simulink model "Autopilot_q_full_5may_new1"  (R2020a)
settings: Solver=ode4  StartTime=0.0  StopTime=300  FixedStep=0.01  RelTol=1e-3
undefined symbols (not defined in the file or in its folder): Aero_cofficients, Atmosphere_pert, Atmospheric_model, Counter_sensor_model, Earth, error_global, flags_global, Guidance_Flags_global, INT_global, param_guidance, Payload_data, Plane_state_mode_finish_catcher_ftr_mode, Plane_state_mode_finish_catcher_fw_mode, Plane_state_mode_finish_catcher_q_mode, Plane_state_mode_finish_catcher_rtr_mode, Plane_state_store, propulsion_model, propulsion_model_int, Structural_data, Thrust_data_store, time_global, WGS84, Wind_data, Wind_model_int, Wind_pert_factor
libraries: simulink x33, aerolibactuator x15, cstblocks x3, aerolibatmos2 x2, aerolibfltsims x1, aerolibtransform2 x1, shared6dof x1
(part 2 of 10)

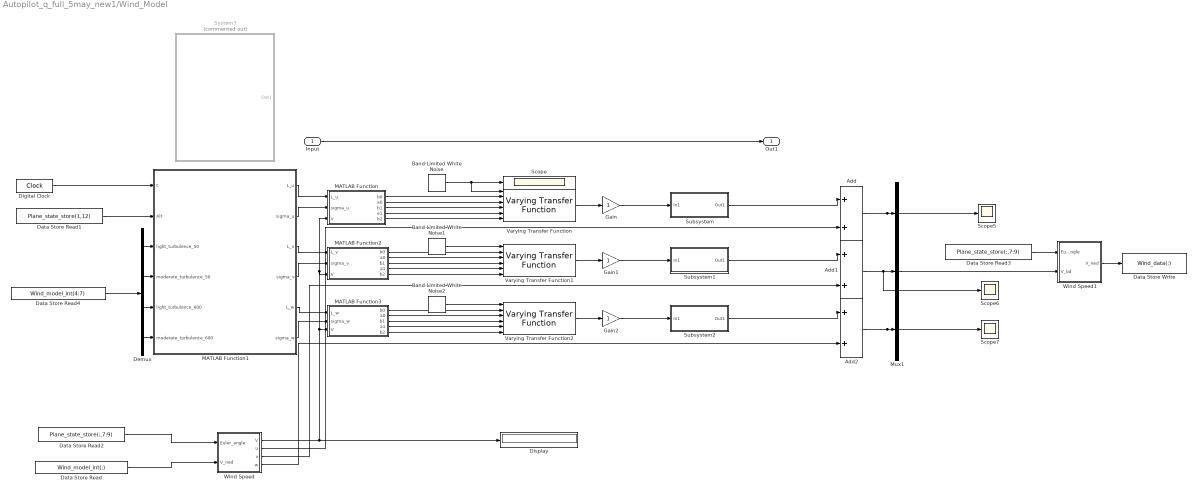
== system Autopilot_q_full_5may_new1/Wind_Model ==
  Input : Inport
  Add : Sum
  Add1 : Sum
  Add2 : Sum
  Band-Limited White Noise : simulink/Sources/Band-Limited White Noise  Cov=[0.001]  Ts=0.01  seed=[23341]
  Band-Limited White Noise1 : simulink/Sources/Band-Limited White Noise  Cov=[0.001]  Ts=0.01  seed=[23341]
  Band-Limited White Noise2 : simulink/Sources/Band-Limited White Noise  Cov=[0.001]  Ts=0.01  seed=[23341]
  Data Store Read : DataStoreRead  DataStoreName=Wind_model_int  SampleTime=0.01  DataStoreElements=Wind_model_int(:)
  Data Store Read1 : DataStoreRead  DataStoreName=Plane_state_store  SampleTime=0.01  DataStoreElements=Plane_state_store(1,12)
  Data Store Read2 : DataStoreRead  DataStoreName=Plane_state_store  SampleTime=0.01  DataStoreElements=Plane_state_store(:,7:9)
  Data Store Read3 : DataStoreRead  DataStoreName=Plane_state_store  DataStoreElements=Plane_state_store(:,7:9)
  Data Store Read4 : DataStoreRead  DataStoreName=Wind_model_int  SampleTime=0.01  DataStoreElements=Wind_model_int(4:7)
  Data Store Write : DataStoreWrite  DataStoreName=Wind_data  SampleTime=0.01  DataStoreElements=Wind_data(:)
  Demux : Demux
  Digital Clock : DigitalClock  SampleTime=0.01
  Display : Display
  Gain : Gain
  Gain1 : Gain
  Gain2 : Gain
  MATLAB Function : MATLAB Function  TreatAsAtomicUnit=on
  MATLAB Function1 : MATLAB Function  TreatAsAtomicUnit=on
  MATLAB Function2 : MATLAB Function  TreatAsAtomicUnit=on
  MATLAB Function3 : MATLAB Function  TreatAsAtomicUnit=on
  Mux1 : Mux  Inputs=3
  Scope{,5..7} (4 alike) : Scope
  Subsystem : Subsystem
  Subsystem1 : Subsystem
  Subsystem2 : Subsystem
  System3 : Subsystem  Commented=on
  Varying Transfer Function : cstblocks/Linear Parameter Varying/Varying Transfer Function  N=2
  Varying Transfer Function1 : cstblocks/Linear Parameter Varying/Varying Transfer Function  N=2
  Varying Transfer Function2 : cstblocks/Linear Parameter Varying/Varying Transfer Function  N=2
  Wind Speed : MATLAB Function  TreatAsAtomicUnit=on
  Wind Speed1 : MATLAB Function  TreatAsAtomicUnit=on  SystemSampleTime=0.01
  Out1 : Outport  VectorParamsAs1DForOutWhenUnconnected=off
  wires:
  Input/1 -> Out1/1
  Demux/3 -> MATLAB Function1/5(light_turbulence_600)
  Demux/1 -> MATLAB Function1/3(light_turbulence_50)
  MATLAB Function1/6(sigma_w) -> MATLAB Function3/2(sigma_w)
  MATLAB Function2/1(b0) -> Varying Transfer Function1/2
  Data Store Read4/1 -> Demux/1
  Band-Limited White Noise/1 -> Varying Transfer Function/1, Scope/1
  MATLAB Function1/4(sigma_v) -> MATLAB Function2/2(sigma_v)
  MATLAB Function1/2(sigma_u) -> MATLAB Function/2(sigma_u)
  MATLAB Function/3(b1) -> Varying Transfer Function/4
  Add1/1 -> Scope6/1, Mux1/2
  Wind Speed/3(v) -> Add1/2
  MATLAB Function2/2(a0) -> Varying Transfer Function1/3
  Mux1/1 -> Wind Speed1/2(V_bd)
  MATLAB Function3/5(b2) -> Varying Transfer Function2/6
  MATLAB Function2/4(a1) -> Varying Transfer Function1/5
  MATLAB Function1/5(L_w) -> MATLAB Function3/1(L_w)
  Data Store Read1/1 -> MATLAB Function1/2(Alt)
  Add2/1 -> Scope7/1, Mux1/3
  Digital Clock/1 -> MATLAB Function1/1(t)
  MATLAB Function3/3(b1) -> Varying Transfer Function2/4
  MATLAB Function3/4(a1) -> Varying Transfer Function2/5
  MATLAB Function/4(a1) -> Varying Transfer Function/5
  MATLAB Function3/2(a0) -> Varying Transfer Function2/3
  Band-Limited White Noise1/1 -> Varying Transfer Function1/1
  Wind Speed1/1(V_ned) -> Data Store Write/1
  Add/1 -> Scope5/1, Mux1/1
  MATLAB Function3/1(b0) -> Varying Transfer Function2/2
  Gain2/1 -> Subsystem2/1(In1)
  Wind Speed/2(u) -> Add/2
  Gain1/1 -> Subsystem1/1(In1)
  Varying Transfer Function/1 -> Gain/1
  Data Store Read2/1 -> Wind Speed/1(Euler_angle)
  Band-Limited White Noise2/1 -> Varying Transfer Function2/1
  Gain/1 -> Subsystem/1(In1)
  Data Store Read3/1 -> Wind Speed1/1(Euler_angle)
  MATLAB Function2/5(b2) -> Varying Transfer Function1/6
  Varying Transfer Function1/1 -> Gain1/1
  MATLAB Function2/3(b1) -> Varying Transfer Function1/4
  MATLAB Function/5(b2) -> Varying Transfer Function/6
  Demux/4 -> MATLAB Function1/6(moderate_turbulence_600)
  MATLAB Function/1(b0) -> Varying Transfer Function/2
  MATLAB Function1/1(L_u) -> MATLAB Function/1(L_u)
  Varying Transfer Function2/1 -> Gain2/1
  MATLAB Function/2(a0) -> Varying Transfer Function/3
  Wind Speed/4(w) -> Add2/2
  Data Store Read/1 -> Wind Speed/2(V_ned)
  Demux/2 -> MATLAB Function1/4(moderate_turbulence_50)
  Wind Speed/1(V) -> MATLAB Function/3(V), MATLAB Function2/3(V), MATLAB Function3/3(V), Display/1
  MATLAB Function1/3(L_v) -> MATLAB Function2/1(L_v)
  Subsystem/1(Out1) -> Add/1
  Subsystem1/1(Out1) -> Add1/1
  Subsystem2/1(Out1) -> Add2/1

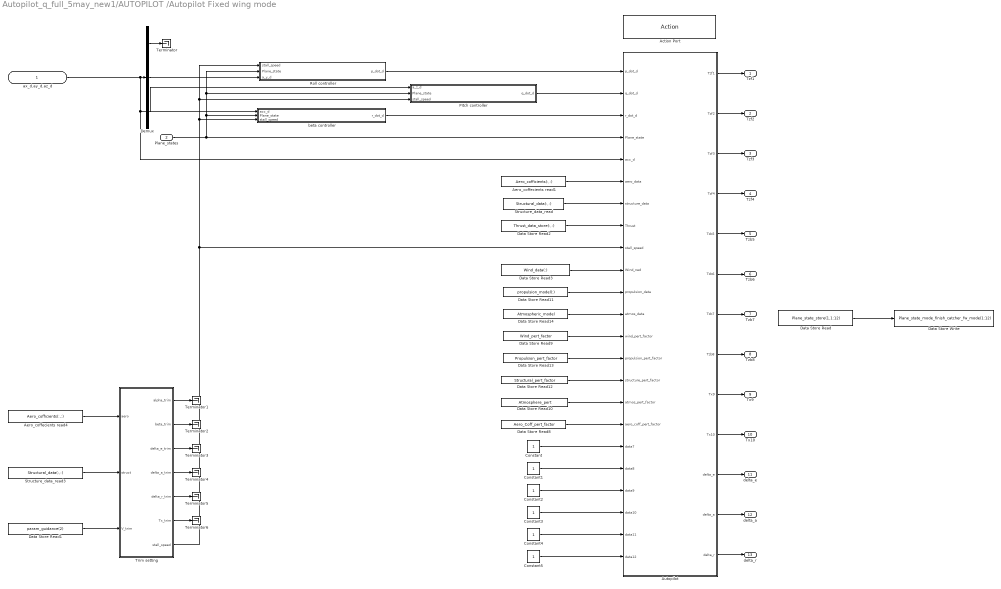
== system Autopilot_q_full_5may_new1/AUTOPILOT /Autopilot Fixed wing mode ==
  ax_d,ay_d,az_d : Inport
  Plane_states : Inport  Port=2
  Action Port : ActionPort  ActionPortLabel=elseif { }
  Aero_coffecients read1 : DataStoreRead  DataStoreName=Aero_cofficients  DataStoreElements=Aero_cofficients(:,:)
  Aero_coffecients read4 : DataStoreRead  DataStoreName=Aero_cofficients  DataStoreElements=Aero_cofficients(:,:)
  Autopilot : MATLAB Function  TreatAsAtomicUnit=on
  Constant{,1..5} (6 alike) : Constant
  Data Store Read : DataStoreRead  DataStoreName=Plane_state_store  DataStoreElements=Plane_state_store(1,1:12)
  Data Store Read1 : DataStoreRead  DataStoreName=param_guidance  DataStoreElements=param_guidance(2)
  Data Store Read10 : DataStoreRead  DataStoreName=Atmosphere_pert
  Data Store Read11 : DataStoreRead  DataStoreName=propulsion_model  DataStoreElements=propulsion_model(:)
  Data Store Read12 : DataStoreRead  DataStoreName=Structural_pert_factor
  Data Store Read13 : DataStoreRead  DataStoreName=Propulsion_pert_factor
  Data Store Read14 : DataStoreRead  DataStoreName=Atmospheric_model
  Data Store Read2 : DataStoreRead  DataStoreName=Thrust_data_store  DataStoreElements=Thrust_data_store(:,:)
  Data Store Read3 : DataStoreRead  DataStoreName=Wind_data  DataStoreElements=Wind_data(:)
  Data Store Read8 : DataStoreRead  DataStoreName=Aero_Coff_pert_factor
  Data Store Read9 : DataStoreRead  DataStoreName=Wind_pert_factor
  Data Store Write : DataStoreWrite  DataStoreName=Plane_state_mode_finish_catcher_fw_mode  DataStoreElements=Plane_state_mode_finish_catcher_fw_mode(1:12)
  Demux : Demux  Outputs=3
  Pitch controller : Subsystem
  Roll controller : Subsystem
  Structure_data_read : DataStoreRead  DataStoreName=Structural_data  DataStoreElements=Structural_data(:,:)
  Structure_data_read3 : DataStoreRead  DataStoreName=Structural_data  DataStoreElements=Structural_data(:,:)
  Terminator{,1..6} (7 alike) : Terminator
  Trim setting : Subsystem
  beta controller : Subsystem
  Tzf1 : Outport  VectorParamsAs1DForOutWhenUnconnected=off
  Tzf2 : Outport  Port=2  VectorParamsAs1DForOutWhenUnconnected=off
  Tzf3 : Outport  Port=3  VectorParamsAs1DForOutWhenUnconnected=off
  Tzf4 : Outport  Port=4  VectorParamsAs1DForOutWhenUnconnected=off
  Tzb5 : Outport  Port=5  VectorParamsAs1DForOutWhenUnconnected=off
  Tzb6 : Outport  Port=6  VectorParamsAs1DForOutWhenUnconnected=off
  Tzb7 : Outport  Port=7  VectorParamsAs1DForOutWhenUnconnected=off
  Tzb8 : Outport  Port=8  VectorParamsAs1DForOutWhenUnconnected=off
  Tx9 : Outport  Port=9  VectorParamsAs1DForOutWhenUnconnected=off
  Tx10 : Outport  Port=10  VectorParamsAs1DForOutWhenUnconnected=off
  delta_e : Outport  Port=11  VectorParamsAs1DForOutWhenUnconnected=off
  delta_a : Outport  Port=12  VectorParamsAs1DForOutWhenUnconnected=off
  delta_r : Outport  Port=13  VectorParamsAs1DForOutWhenUnconnected=off
  wires:
  beta controller/1(r_dot_d) -> Autopilot/3(r_dot_d)
  Trim setting/5(delta_r_trim) -> Terminator5/1
  Autopilot/8(Tzb8) -> Tzb8/1
  Autopilot/4(Tzf4) -> Tzf4/1
  Autopilot/1(Tzf1) -> Tzf1/1
  Data Store Read1/1 -> Trim setting/3(V_trim)
  Structure_data_read3/1 -> Trim setting/2("struct ")
  Autopilot/2(Tzf2) -> Tzf2/1
  Trim setting/4(delta_a_trim) -> Terminator4/1
  Autopilot/10(Tx10) -> Tx10/1
  Trim setting/3(delta_e_trim) -> Terminator3/1
  Structure_data_read/1 -> Autopilot/7(structure_data)
  Roll controller/1(p_dot_d) -> Autopilot/1(p_dot_d)
  Autopilot/3(Tzf3) -> Tzf3/1
  Autopilot/9(Tx9) -> Tx9/1
  Data Store Read2/1 -> Autopilot/8(Thrust)
  Trim setting/6(Tx_trim) -> Terminator6/1
  Autopilot/6(Tzb6) -> Tzb6/1
  Autopilot/13(delta_r) -> delta_r/1
  Trim setting/2(beta_trim) -> Terminator2/1
  Aero_coffecients read1/1 -> Autopilot/6(aero_data)
  Autopilot/12(delta_a) -> delta_a/1
  Autopilot/7(Tzb7) -> Tzb7/1
  Autopilot/11(delta_e) -> delta_e/1
  Trim setting/7(stall_speed) -> Autopilot/9(stall_speed), beta controller/3(stall_speed), Roll controller/1(stall_speed), Pitch controller/3(stall_speed)
  Aero_coffecients read4/1 -> Trim setting/1("aero ")
  Autopilot/5(Tzb5) -> Tzb5/1
  Trim setting/1(alpha_trim) -> Terminator1/1
  Pitch controller/1(q_dot_d) -> Autopilot/2(q_dot_d)
  Data Store Read/1 -> Data Store Write/1
  ax_d,ay_d,az_d/1 -> Autopilot/5(acc_d), beta controller/1(acc_d), Demux/1
  Demux/3 -> Pitch controller/1(a_z_d)
  Demux/2 -> Roll controller/3(a_y_d)
  Demux/1 -> Terminator/1
  Plane_states/1 -> Pitch controller/2(Plane_state), Roll controller/2(Plane_state), beta controller/2(Plane_state), Autopilot/4(Plane_state)
  Data Store Read3/1 -> Autopilot/10(Wind_ned)
  Data Store Read11/1 -> Autopilot/11(propulsion_data)
  Data Store Read14/1 -> Autopilot/12(atmos_data)
  Data Store Read9/1 -> Autopilot/13(wind_pert_factor)
  Data Store Read13/1 -> Autopilot/14(propulsion_pert_factor)
  Data Store Read12/1 -> Autopilot/15(structure_pert_factor)
  Data Store Read10/1 -> Autopilot/16(atmos_pert_factor)
  Data Store Read8/1 -> Autopilot/17(aero_coff_pert_factor)
  Constant/1 -> Autopilot/18(data7)
  Constant1/1 -> Autopilot/19(data8)
  Constant2/1 -> Autopilot/20(data9)
  Constant3/1 -> Autopilot/21(data10)
  Constant4/1 -> Autopilot/22(data11)
  Constant5/1 -> Autopilot/23(data12)

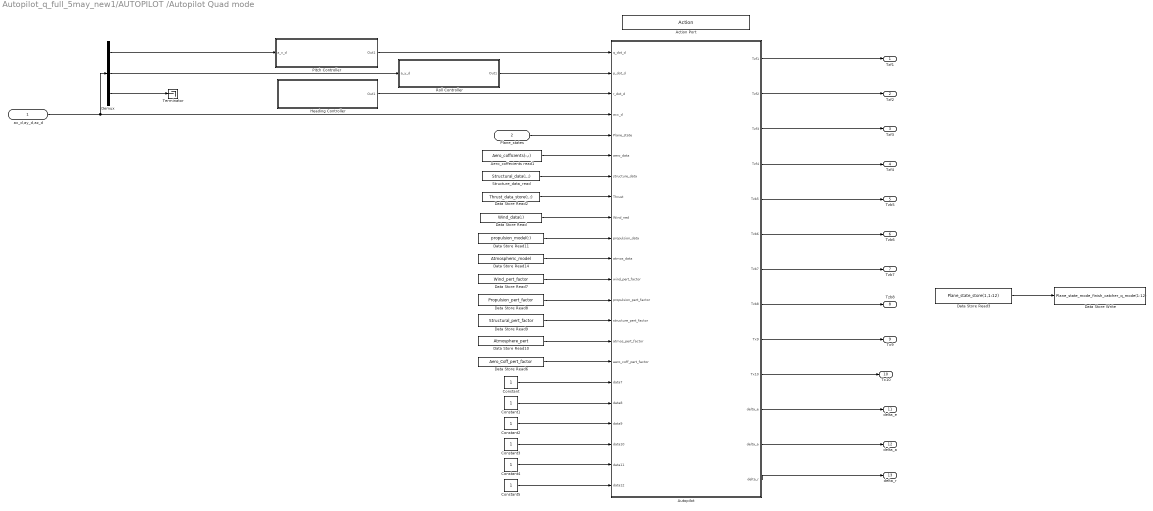
== system Autopilot_q_full_5may_new1/AUTOPILOT /Autopilot Quad mode ==
  ax_d,ay_d,az_d : Inport
  Plane_states : Inport  Port=2
  Action Port : ActionPort  ActionPortLabel=if { }
  Aero_coffecients read1 : DataStoreRead  DataStoreName=Aero_cofficients  DataStoreElements=Aero_cofficients(:,:)
  Autopilot : MATLAB Function  TreatAsAtomicUnit=on
  Constant{,1..5} (6 alike) : Constant
  Data Store Read : DataStoreRead  DataStoreName=Wind_data  DataStoreElements=Wind_data(:)
  Data Store Read10 : DataStoreRead  DataStoreName=Atmosphere_pert
  Data Store Read11 : DataStoreRead  DataStoreName=propulsion_model  DataStoreElements=propulsion_model(:)
  Data Store Read14 : DataStoreRead  DataStoreName=Atmospheric_model
  Data Store Read2 : DataStoreRead  DataStoreName=Thrust_data_store  DataStoreElements=Thrust_data_store(:,:)
  Data Store Read3 : DataStoreRead  DataStoreName=Plane_state_store  DataStoreElements=Plane_state_store(1,1:12)
  Data Store Read6 : DataStoreRead  DataStoreName=Aero_Coff_pert_factor
  Data Store Read7 : DataStoreRead  DataStoreName=Wind_pert_factor
  Data Store Read8 : DataStoreRead  DataStoreName=Propulsion_pert_factor
  Data Store Read9 : DataStoreRead  DataStoreName=Structural_pert_factor
  Data Store Write : DataStoreWrite  DataStoreName=Plane_state_mode_finish_catcher_q_mode  DataStoreElements=Plane_state_mode_finish_catcher_q_mode(1:12)
  Demux : Demux  Outputs=3
  Heading Controller : Subsystem
  Pitch Controller : Subsystem
  Roll Controller : Subsystem
  Structure_data_read : DataStoreRead  DataStoreName=Structural_data  DataStoreElements=Structural_data(:,:)
  Terminator : Terminator
  Tzf1 : Outport  VectorParamsAs1DForOutWhenUnconnected=off
  Tzf2 : Outport  Port=2  VectorParamsAs1DForOutWhenUnconnected=off
  Tzf3 : Outport  Port=3  VectorParamsAs1DForOutWhenUnconnected=off
  Tzf4 : Outport  Port=4  VectorParamsAs1DForOutWhenUnconnected=off
  Tzb5 : Outport  Port=5  VectorParamsAs1DForOutWhenUnconnected=off
  Tzb6 : Outport  Port=6  VectorParamsAs1DForOutWhenUnconnected=off
  Tzb7 : Outport  Port=7  VectorParamsAs1DForOutWhenUnconnected=off
  Tzb8 : Outport  Port=8  VectorParamsAs1DForOutWhenUnconnected=off
  Tx9 : Outport  Port=9  VectorParamsAs1DForOutWhenUnconnected=off
  Tx10 : Outport  Port=10  VectorParamsAs1DForOutWhenUnconnected=off
  delta_e : Outport  Port=11  VectorParamsAs1DForOutWhenUnconnected=off
  delta_a : Outport  Port=12  VectorParamsAs1DForOutWhenUnconnected=off
  delta_r : Outport  Port=13  VectorParamsAs1DForOutWhenUnconnected=off
  wires:
  Data Store Read2/1 -> Autopilot/8(Thrust)
  Aero_coffecients read1/1 -> Autopilot/6(aero_data)
  Autopilot/13(delta_r) -> delta_r/1
  Autopilot/7(Tzb7) -> Tzb7/1
  Structure_data_read/1 -> Autopilot/7(structure_data)
  Autopilot/4(Tzf4) -> Tzf4/1
  Autopilot/12(delta_a) -> delta_a/1
  Autopilot/5(Tzb5) -> Tzb5/1
  Autopilot/11(delta_e) -> delta_e/1
  Autopilot/3(Tzf3) -> Tzf3/1
  Plane_states/1 -> Autopilot/5(Plane_state)
  Autopilot/6(Tzb6) -> Tzb6/1
  Autopilot/9(Tx9) -> Tx9/1
  Autopilot/1(Tzf1) -> Tzf1/1
  Autopilot/2(Tzf2) -> Tzf2/1
  Autopilot/10(Tx10) -> Tx10/1
  Autopilot/8(Tzb8) -> Tzb8/1
  ax_d,ay_d,az_d/1 -> Autopilot/4(acc_d), Demux/1
  Demux/3 -> Terminator/1
  Data Store Read3/1 -> Data Store Write/1
  Demux/1 -> Pitch Controller/1(a_x_d)
  Demux/2 -> Roll Controller/1(a_y_d)
  Heading Controller/1(Out1) -> Autopilot/3(r_dot_d)
  Pitch Controller/1(Out1) -> Autopilot/1(q_dot_d)
  Roll Controller/1(Out1) -> Autopilot/2(p_dot_d)
  Data Store Read/1 -> Autopilot/9(Wind_ned)
  Data Store Read11/1 -> Autopilot/10(propulsion_data)
  Data Store Read14/1 -> Autopilot/11(atmos_data)
  Data Store Read6/1 -> Autopilot/16(aero_coff_pert_factor)
  Data Store Read7/1 -> Autopilot/12(wind_pert_factor)
  Data Store Read8/1 -> Autopilot/13(propulsion_pert_factor)
  Data Store Read9/1 -> Autopilot/14(structure_pert_factor)
  Data Store Read10/1 -> Autopilot/15(atmos_pert_factor)
  Constant4/1 -> Autopilot/21(data11)
  Constant3/1 -> Autopilot/20(data10)
  Constant2/1 -> Autopilot/19(data9)
  Constant1/1 -> Autopilot/18(data8)
  Constant/1 -> Autopilot/17(data7)
  Constant5/1 -> Autopilot/22(data12)

== system Autopilot_q_full_5may_new1/AUTOPILOT /Autopilot Transition mode ==
  ax,ay,az : Inport
  Plane_state : Inport  Port=2
  Action Port : ActionPort  ActionPortLabel=elseif { }
  Data Store Read : DataStoreRead  DataStoreName=flags_global  DataStoreElements=flags_global(23)
  Data Store Read1 : DataStoreRead  DataStoreName=flags_global  DataStoreElements=flags_global(24)
  Data Store Read2 : DataStoreRead  DataStoreName=Thrust_data_store  DataStoreElements=Thrust_data_store(:,:)
  Demux : Demux  Outputs=13
  Forward transition : Subsystem
  If : If  IfExpression=u1 ==1  ShowElse=off
  If1 : If  IfExpression=u1 ==1  ShowElse=off
  Mux : Mux  Inputs=13
  Mux1 : Mux  Inputs=13
  Reverse transition : Subsystem
  Switch1 : Switch  Criteria=u2 ~= 0
  Tzf1 : Outport  VectorParamsAs1DForOutWhenUnconnected=off
  Tzf2 : Outport  Port=2  VectorParamsAs1DForOutWhenUnconnected=off
  Tzf3 : Outport  Port=3  VectorParamsAs1DForOutWhenUnconnected=off
  Tzf4 : Outport  Port=4  VectorParamsAs1DForOutWhenUnconnected=off
  Tzb5 : Outport  Port=5  VectorParamsAs1DForOutWhenUnconnected=off
  Tzb6 : Outport  Port=6  VectorParamsAs1DForOutWhenUnconnected=off
  Tzb7 : Outport  Port=7  VectorParamsAs1DForOutWhenUnconnected=off
  Tzb8 : Outport  Port=8  VectorParamsAs1DForOutWhenUnconnected=off
  Tx9 : Outport  Port=9  VectorParamsAs1DForOutWhenUnconnected=off
  Tx10 : Outport  Port=10  VectorParamsAs1DForOutWhenUnconnected=off
  delta_e : Outport  Port=11  VectorParamsAs1DForOutWhenUnconnected=off
  delta_a : Outport  Port=12  VectorParamsAs1DForOutWhenUnconnected=off
  delta_r : Outport  Port=13  VectorParamsAs1DForOutWhenUnconnected=off
  wires:
  ax,ay,az/1 -> Reverse transition/1(ax_d,ay_d,az_d), Forward transition/1(ax_d,ay_d,az_d)
  Plane_state/1 -> Forward transition/2(Plane_states), Reverse transition/2(Plane_states)
  Forward transition/1(Tzf1) -> Mux/1
  Forward transition/2(Tzf2) -> Mux/2
  Forward transition/3(Tzf3) -> Mux/3
  Forward transition/4(Tzf4) -> Mux/4
  Forward transition/5(Tzb5) -> Mux/5
  Forward transition/6(Tzb6) -> Mux/6
  Forward transition/7(Tzb7) -> Mux/7
  Forward transition/8(Tzb8) -> Mux/8
  Forward transition/9(Tx9) -> Mux/9
  Forward transition/10(Tx10) -> Mux/10
  Forward transition/11(delta_e) -> Mux/11
  Forward transition/12(delta_a) -> Mux/12
  Forward transition/13(delta_r) -> Mux/13
  Reverse transition/1(Tzf1) -> Mux1/1
  Reverse transition/2(Tzf2) -> Mux1/2
  Reverse transition/3(Tzf3) -> Mux1/3
  Reverse transition/4(Tzf4) -> Mux1/4
  Reverse transition/5(Tzb5) -> Mux1/5
  Reverse transition/6(Tzb6) -> Mux1/6
  Reverse transition/7(Tzb7) -> Mux1/7
  Reverse transition/8(Tzb8) -> Mux1/8
  Reverse transition/9(Tx9) -> Mux1/9
  Reverse transition/10(Tx10) -> Mux1/10
  Reverse transition/11(delta_e) -> Mux1/11
  Reverse transition/12(delta_a) -> Mux1/12
  Reverse transition/13(delta_r) -> Mux1/13
  Switch1/1 -> Demux/1
  Mux/1 -> Switch1/1
  Mux1/1 -> Switch1/3
  Demux/1 -> Tzf1/1
  Demux/2 -> Tzf2/1
  Demux/3 -> Tzf3/1
  Demux/4 -> Tzf4/1
  Demux/5 -> Tzb5/1
  Demux/6 -> Tzb6/1
  Demux/7 -> Tzb7/1
  Demux/8 -> Tzb8/1
  Demux/9 -> Tx9/1
  Demux/10 -> Tx10/1
  Demux/11 -> delta_e/1
  Demux/12 -> delta_a/1
  Demux/13 -> delta_r/1
  Data Store Read1/1 -> If1/1
  Data Store Read/1 -> If/1, Switch1/2
  Data Store Read2/1 -> Forward transition/3(Thrust), Reverse transition/3(Thrust)
  If1/1 -> Reverse transition/Action
  If/1 -> Forward transition/Action

== system Autopilot_q_full_5may_new1/AUTOPILOT /Subsystem ==
  In1 : Inport  SampleTime=0.01
  In2 : Inport  Port=2  SampleTime=0.01
  In3 : Inport  Port=3  SampleTime=0.01
  Out1 : Outport  VectorParamsAs1DForOutWhenUnconnected=off
  Out2 : Outport  Port=2  VectorParamsAs1DForOutWhenUnconnected=off
  Out3 : Outport  Port=3  VectorParamsAs1DForOutWhenUnconnected=off
  wires:
  In1/1 -> Out1/1
  In2/1 -> Out2/1
  In3/1 -> Out3/1

== system Autopilot_q_full_5may_new1/All SENSOR MODEL2/INS BODY RATES ==
  In3 : Inport
  In4 : Inport  Port=2
  Clock1 : Clock
  Data Store Read2 : DataStoreRead  DataStoreName=Counter_sensor_model  DataStoreElements=Counter_sensor_model(2)
  Data Store Read3 : DataStoreRead  DataStoreName=Counter_sensor_model  DataStoreElements=Counter_sensor_model(6)
  Data Store Read4 : DataStoreRead  DataStoreName=Plane_state_store  DataStoreElements=Plane_state_store(:,4:6)
  Data Store Write1 : DataStoreWrite  DataStoreName=Counter_sensor_model  DataStoreElements=Counter_sensor_model(2)
  Data Store Write2 : DataStoreWrite  DataStoreName=Counter_sensor_model  DataStoreElements=Counter_sensor_model(6)
  Demux : Demux  Outputs=3
  Demux1 : Demux  Outputs=3
  MATLAB Function2 : MATLAB Function
  Scope : Scope
  Out1 : Outport  VectorParamsAs1DForOutWhenUnconnected=off
  Out3 : Outport  Port=2  VectorParamsAs1DForOutWhenUnconnected=off
  Out4 : Outport  Port=3  VectorParamsAs1DForOutWhenUnconnected=off
  wires:
  Data Store Read4/1 -> MATLAB Function2/6(in_old)
  MATLAB Function2/1(count_temp) -> Data Store Write2/1
  Clock1/1 -> MATLAB Function2/1(t)
  Data Store Read3/1 -> MATLAB Function2/8("count_temp ")
  Demux1/2 -> MATLAB Function2/3(frequency_imu)
  Demux1/3 -> MATLAB Function2/4(frequency_nav)
  In4/1 -> MATLAB Function2/5(in)
  In3/1 -> Demux1/1
  MATLAB Function2/2(count) -> Data Store Write1/1, Scope/1
  Data Store Read2/1 -> MATLAB Function2/7("count ")
  Demux1/1 -> MATLAB Function2/2(frequency_plant)
  MATLAB Function2/3(y) -> Demux/1
  Demux/2 -> Out3/1
  Demux/1 -> Out1/1
  Demux/3 -> Out4/1

== system Autopilot_q_full_5may_new1/All SENSOR MODEL2/INS EULER ANGLE ==
  In3 : Inport
  In4 : Inport  Port=2
  Clock1 : Clock
  Data Store Read2 : DataStoreRead  DataStoreName=Counter_sensor_model  DataStoreElements=Counter_sensor_model(3)
  Data Store Read3 : DataStoreRead  DataStoreName=Counter_sensor_model  DataStoreElements=Counter_sensor_model(7)
  Data Store Read4 : DataStoreRead  DataStoreName=Plane_state_store  DataStoreElements=Plane_state_store(:,7:9)
  Data Store Write1 : DataStoreWrite  DataStoreName=Counter_sensor_model  DataStoreElements=Counter_sensor_model(3)
  Data Store Write2 : DataStoreWrite  DataStoreName=Counter_sensor_model  DataStoreElements=Counter_sensor_model(7)
  Demux : Demux  Outputs=3
  Demux1 : Demux  Outputs=3
  MATLAB Function2 : MATLAB Function
  Scope : Scope
  Out1 : Outport  VectorParamsAs1DForOutWhenUnconnected=off
  Out2 : Outport  Port=2  VectorParamsAs1DForOutWhenUnconnected=off
  Out3 : Outport  Port=3  VectorParamsAs1DForOutWhenUnconnected=off
  wires:
  Demux1/1 -> MATLAB Function2/2(frequency_plant)
  Data Store Read2/1 -> MATLAB Function2/7("count ")
  MATLAB Function2/2(count) -> Scope/1, Data Store Write1/1
  In3/1 -> Demux1/1
  In4/1 -> MATLAB Function2/5(in)
  Demux1/3 -> MATLAB Function2/4(frequency_nav)
  Demux1/2 -> MATLAB Function2/3(frequency_imu)
  Data Store Read3/1 -> MATLAB Function2/8("count_temp ")
  Clock1/1 -> MATLAB Function2/1(t)
  MATLAB Function2/1(count_temp) -> Data Store Write2/1
  Data Store Read4/1 -> MATLAB Function2/6(in_old)
  MATLAB Function2/3(y) -> Demux/1
  Demux/2 -> Out2/1
  Demux/1 -> Out1/1
  Demux/3 -> Out3/1

== system Autopilot_q_full_5may_new1/All SENSOR MODEL2/INS NAV POSITION ==
  In3 : Inport
  In4 : Inport  Port=2
  Clock1 : Clock
  Data Store Read2 : DataStoreRead  DataStoreName=Counter_sensor_model  DataStoreElements=Counter_sensor_model(4)
  Data Store Read3 : DataStoreRead  DataStoreName=Counter_sensor_model  DataStoreElements=Counter_sensor_model(8)
  Data Store Read4 : DataStoreRead  DataStoreName=Plane_state_store  DataStoreElements=Plane_state_store(:,10:12)
  Data Store Write1 : DataStoreWrite  DataStoreName=Counter_sensor_model  DataStoreElements=Counter_sensor_model(4)
  Data Store Write2 : DataStoreWrite  DataStoreName=Counter_sensor_model  DataStoreElements=Counter_sensor_model(8)
  Demux : Demux  Outputs=3
  Demux1 : Demux  Outputs=3
  MATLAB Function2 : MATLAB Function
      settings: MinAlgLoopOccurrences=on
  Scope : Scope
  Out1 : Outport  VectorParamsAs1DForOutWhenUnconnected=off
  Out3 : Outport  Port=2  VectorParamsAs1DForOutWhenUnconnected=off
  Out4 : Outport  Port=3  VectorParamsAs1DForOutWhenUnconnected=off
  wires:
  Data Store Read4/1 -> MATLAB Function2/6(in_old)
  MATLAB Function2/1(count_temp) -> Data Store Write2/1
  Clock1/1 -> MATLAB Function2/1(t)
  Data Store Read3/1 -> MATLAB Function2/8("count_temp ")
  Demux1/2 -> MATLAB Function2/3(frequency_imu)
  Demux1/3 -> MATLAB Function2/4(frequency_nav)
  In4/1 -> MATLAB Function2/5(in)
  In3/1 -> Demux1/1
  MATLAB Function2/2(count) -> Data Store Write1/1, Scope/1
  Data Store Read2/1 -> MATLAB Function2/7("count ")
  Demux1/1 -> MATLAB Function2/2(frequency_plant)
  MATLAB Function2/3(y) -> Demux/1
  Demux/2 -> Out3/1
  Demux/1 -> Out1/1
  Demux/3 -> Out4/1

== system Autopilot_q_full_5may_new1/All SENSOR MODEL2/INS NAV VELOCITY   ==
  In3 : Inport
  In4 : Inport  Port=2
  Clock1 : Clock
  Data Store Read2 : DataStoreRead  DataStoreName=Counter_sensor_model  DataStoreElements=Counter_sensor_model(1)
  Data Store Read3 : DataStoreRead  DataStoreName=Counter_sensor_model  DataStoreElements=Counter_sensor_model(5)
  Data Store Read4 : DataStoreRead  DataStoreName=Plane_state_store  DataStoreElements=Plane_state_store(1,1:3)
  Data Store Write1 : DataStoreWrite  DataStoreName=Counter_sensor_model  DataStoreElements=Counter_sensor_model(1)
  Data Store Write2 : DataStoreWrite  DataStoreName=Counter_sensor_model  DataStoreElements=Counter_sensor_model(5)
  Demux : Demux  Outputs=3
  Demux1 : Demux  Outputs=3
  MATLAB Function2 : MATLAB Function
  Scope : Scope
  Out1 : Outport  VectorParamsAs1DForOutWhenUnconnected=off
  Out2 : Outport  Port=2  VectorParamsAs1DForOutWhenUnconnected=off
  Out3 : Outport  Port=3  VectorParamsAs1DForOutWhenUnconnected=off
  wires:
  Demux1/1 -> MATLAB Function2/2(frequency_plant)
  Data Store Read2/1 -> MATLAB Function2/7("count ")
  MATLAB Function2/2(count) -> Data Store Write1/1, Scope/1
  In3/1 -> Demux1/1
  In4/1 -> MATLAB Function2/5(in)
  MATLAB Function2/3(y) -> Demux/1
  Demux1/3 -> MATLAB Function2/4(frequency_nav)
  Demux1/2 -> MATLAB Function2/3(frequency_imu)
  Data Store Read3/1 -> MATLAB Function2/8("count_temp ")
  Clock1/1 -> MATLAB Function2/1(t)
  MATLAB Function2/1(count_temp) -> Data Store Write2/1
  Data Store Read4/1 -> MATLAB Function2/6(in_old)
  Demux/1 -> Out1/1
  Demux/2 -> Out2/1
  Demux/3 -> Out3/1

== system Autopilot_q_full_5may_new1/Battery Model/Subsystem ==
  note: Modified Battery Capacity
  In1 : Inport
  Out1 : Outport  VectorParamsAs1DForOutWhenUnconnected=off
  wires:
  In1/1 -> Out1/1

== system Autopilot_q_full_5may_new1/INITIALISE_PARAMS/INITIALISE MODELS ==
  In1 : Inport
  Action Port : ActionPort  ActionPortLabel=else { }
  Out1 : Outport  VectorParamsAs1DForOutWhenUnconnected=off
  wires:
  In1/1 -> Out1/1

== system Autopilot_q_full_5may_new1/INITIALISE_PARAMS/If Action Subsystem ==
  note: Params
  note: INT_Global
  note: Error_Global
  note: Aero_Coffecients
  note: Time_Global
  note: Structure_Data
  note: Flags_Global
  note: INITIALISER
  note: Atmos model
  note: Aero_pert
  note: Structure_pert
  note: Wind_pert
  note: Propulsion_pert
  note: Atmosphere_pert
  note: Propulsion model
  note: Wind_Model
  note: Payload_data
  In1 : Inport
  Action Port : ActionPort  ActionPortLabel=if { }
  Aero Cofficients : Subsystem
  Aero_data_perturbation : Subsystem
  Atmosphere_pert : Subsystem
  Atmospheric model : Subsystem
  INT_global : Subsystem
  Params : Subsystem
  Payload_data : Subsystem
  Propulsion_Model : Subsystem
  Propulsion_data_pert : Subsystem
  Structure_data : Subsystem
  Structure_data_pert : Subsystem
  Time_global : Subsystem
  Wind_Model : Subsystem
  Wind_data_pert : Subsystem
  error_global : Subsystem
  flags_global : Subsystem
  Out1 : Outport  VectorParamsAs1DForOutWhenUnconnected=off
  wires:
  In1/1 -> Out1/1

== system Autopilot_q_full_5may_new1/Payload force and moment/Changing Mass ==
  In1 : Inport
  MATLAB Function : MATLAB Function  TreatAsAtomicUnit=on
  Out1 : Outport  VectorParamsAs1DForOutWhenUnconnected=off
  wires:
  In1/1 -> MATLAB Function/1(ideal_Plane_state)
  MATLAB Function/1(mass) -> Out1/1

== system Autopilot_q_full_5may_new1/Plotter/rad2deg ==
  In1 : Inport
  Constant1 : Constant  Value=57.3
  Multiply1 : Product
  Out1 : Outport  VectorParamsAs1DForOutWhenUnconnected=off
  wires:
  Constant1/1 -> Multiply1/1
  In1/1 -> Multiply1/2
  Multiply1/1 -> Out1/1

== system Autopilot_q_full_5may_new1/Plotter/rad2deg1 ==
  In1 : Inport
  Constant1 : Constant  Value=57.3
  Multiply1 : Product
  Out1 : Outport  VectorParamsAs1DForOutWhenUnconnected=off
  wires:
  Multiply1/1 -> Out1/1
  In1/1 -> Multiply1/2
  Constant1/1 -> Multiply1/1

== system Autopilot_q_full_5may_new1/Plotter/rad2deg2 ==
  In1 : Inport
  Constant1 : Constant  Value=57.3
  Multiply1 : Product
  Out1 : Outport  VectorParamsAs1DForOutWhenUnconnected=off
  wires:
  Constant1/1 -> Multiply1/1
  In1/1 -> Multiply1/2
  Multiply1/1 -> Out1/1

== system Autopilot_q_full_5may_new1/Plotter/rad2deg3 ==
  In1 : Inport
  Constant1 : Constant  Value=57.3
  Multiply1 : Product
  Out1 : Outport  VectorParamsAs1DForOutWhenUnconnected=off
  wires:
  Multiply1/1 -> Out1/1
  In1/1 -> Multiply1/2
  Constant1/1 -> Multiply1/1

== system Autopilot_q_full_5may_new1/Plotter/rad2deg4 ==
  In1 : Inport
  Constant1 : Constant  Value=57.3
  Multiply1 : Product
  Out1 : Outport  VectorParamsAs1DForOutWhenUnconnected=off
  wires:
  Constant1/1 -> Multiply1/1
  In1/1 -> Multiply1/2
  Multiply1/1 -> Out1/1

== system Autopilot_q_full_5may_new1/Plotter/rad2deg5 ==
  In1 : Inport
  Constant1 : Constant  Value=57.3
  Multiply1 : Product
  Out1 : Outport  VectorParamsAs1DForOutWhenUnconnected=off
  wires:
  Multiply1/1 -> Out1/1
  In1/1 -> Multiply1/2
  Constant1/1 -> Multiply1/1

== system Autopilot_q_full_5may_new1/Plotter/rad2deg6 ==
  In1 : Inport
  Constant1 : Constant  Value=57.3
  Multiply1 : Product
  Out1 : Outport  VectorParamsAs1DForOutWhenUnconnected=off
  wires:
  Multiply1/1 -> Out1/1
  In1/1 -> Multiply1/2
  Constant1/1 -> Multiply1/1

== system Autopilot_q_full_5may_new1/Plotter/rad2deg7 ==
  In1 : Inport
  Constant1 : Constant  Value=57.3
  Multiply1 : Product
  Out1 : Outport  VectorParamsAs1DForOutWhenUnconnected=off
  wires:
  Constant1/1 -> Multiply1/1
  In1/1 -> Multiply1/2
  Multiply1/1 -> Out1/1

== system Autopilot_q_full_5may_new1/Plotter/rad2deg8 ==
  In1 : Inport
  Constant1 : Constant  Value=57.3
  Multiply1 : Product
  Out1 : Outport  VectorParamsAs1DForOutWhenUnconnected=off
  wires:
  Multiply1/1 -> Out1/1
  In1/1 -> Multiply1/2
  Constant1/1 -> Multiply1/1

== system Autopilot_q_full_5may_new1/Plotter/rad2deg9 ==
  In1 : Inport
  Constant1 : Constant  Value=57.3
  Multiply1 : Product
  Out1 : Outport  VectorParamsAs1DForOutWhenUnconnected=off
  wires:
  Multiply1/1 -> Out1/1
  In1/1 -> Multiply1/2
  Constant1/1 -> Multiply1/1

== system Autopilot_q_full_5may_new1/Plotter/ten_power_neg_5_zerorer ==
  In1 : Inport
  MATLAB Function : MATLAB Function  TreatAsAtomicUnit=on
  Out1 : Outport  VectorParamsAs1DForOutWhenUnconnected=off
  wires:
  In1/1 -> MATLAB Function/1(u)
  MATLAB Function/1(y) -> Out1/1

== system Autopilot_q_full_5may_new1/Plotter/ten_power_neg_5_zerorer1 ==
  In1 : Inport
  MATLAB Function : MATLAB Function  TreatAsAtomicUnit=on
  Out1 : Outport  VectorParamsAs1DForOutWhenUnconnected=off
  wires:
  In1/1 -> MATLAB Function/1(u)
  MATLAB Function/1(y) -> Out1/1

== system Autopilot_q_full_5may_new1/Plotter/ten_power_neg_5_zerorer2 ==
  In1 : Inport
  MATLAB Function : MATLAB Function  TreatAsAtomicUnit=on
  Out1 : Outport  VectorParamsAs1DForOutWhenUnconnected=off
  wires:
  MATLAB Function/1(y) -> Out1/1
  In1/1 -> MATLAB Function/1(u)

== system Autopilot_q_full_5may_new1/Plotter/ten_power_neg_5_zerorer3 ==
  In1 : Inport
  MATLAB Function : MATLAB Function  TreatAsAtomicUnit=on
  Out1 : Outport  VectorParamsAs1DForOutWhenUnconnected=off
  wires:
  In1/1 -> MATLAB Function/1(u)
  MATLAB Function/1(y) -> Out1/1

== system Autopilot_q_full_5may_new1/Plotter/thrust to rpm ==
  motor_para : Inport
  Thrust : Inport  Port=2
  density : Inport  Port=3
  MATLAB Function : MATLAB Function  TreatAsAtomicUnit=on
  RPM : Outport  VectorParamsAs1DForOutWhenUnconnected=off
  wires:
  Thrust/1 -> MATLAB Function/2(u)
  MATLAB Function/1(omega) -> RPM/1
  motor_para/1 -> MATLAB Function/1(motor_para)
  density/1 -> MATLAB Function/3(density)

== system Autopilot_q_full_5may_new1/Wind_Model/Subsystem ==
  In1 : Inport
  Data Store Read1 : DataStoreRead  DataStoreName=Plane_state_store  DataStoreElements=Plane_state_store(1,12)
  Data Store Read5 : DataStoreRead  DataStoreName=Wind_model_int  DataStoreElements=Wind_model_int(:)
  MATLAB Function : MATLAB Function  TreatAsAtomicUnit=on
  Out1 : Outport  VectorParamsAs1DForOutWhenUnconnected=off
  wires:
  In1/1 -> MATLAB Function/1(u)
  MATLAB Function/1(y) -> Out1/1
  Data Store Read5/1 -> MATLAB Function/2(Wind_model_int)
  Data Store Read1/1 -> MATLAB Function/3(Z)

== system Autopilot_q_full_5may_new1/Wind_Model/Subsystem1 ==
  In1 : Inport
  Data Store Read1 : DataStoreRead  DataStoreName=Plane_state_store  DataStoreElements=Plane_state_store(1,12)
  Data Store Read5 : DataStoreRead  DataStoreName=Wind_model_int  DataStoreElements=Wind_model_int(:)
  MATLAB Function : MATLAB Function  TreatAsAtomicUnit=on
  Out1 : Outport  VectorParamsAs1DForOutWhenUnconnected=off
  wires:
  Data Store Read1/1 -> MATLAB Function/3(Z)
  Data Store Read5/1 -> MATLAB Function/2(Wind_model_int)
  MATLAB Function/1(y) -> Out1/1
  In1/1 -> MATLAB Function/1(u)

== system Autopilot_q_full_5may_new1/Wind_Model/Subsystem2 ==
  In1 : Inport
  Data Store Read1 : DataStoreRead  DataStoreName=Plane_state_store  DataStoreElements=Plane_state_store(1,12)
  Data Store Read5 : DataStoreRead  DataStoreName=Wind_model_int  DataStoreElements=Wind_model_int(:)
  MATLAB Function : MATLAB Function  TreatAsAtomicUnit=on
  Out1 : Outport  VectorParamsAs1DForOutWhenUnconnected=off
  wires:
  In1/1 -> MATLAB Function/1(u)
  MATLAB Function/1(y) -> Out1/1
  Data Store Read5/1 -> MATLAB Function/2(Wind_model_int)
  Data Store Read1/1 -> MATLAB Function/3(Z)

== system Autopilot_q_full_5may_new1/Wind_Model/System3 ==
  Add : Sum
  Add1 : Sum
  Add2 : Sum
  Band-Limited White Noise : simulink/Sources/Band-Limited White Noise  Cov=[0.001]  Ts=0.01  seed=[23341]
  Band-Limited White Noise1 : simulink/Sources/Band-Limited White Noise  Cov=[0.001]  Ts=0.01  seed=[23341]
  Band-Limited White Noise2 : simulink/Sources/Band-Limited White Noise  Cov=[0.001]  Ts=0.01  seed=[23341]
  Mux : Mux  Inputs=3
  Mux1 : Mux  Inputs=3
  Scope{1..3,5..7} (6 alike) : Scope
  Subsystem1 : Subsystem  Commented=on
  Subsystem4 : Subsystem  Commented=on
  Subsystem5 : Subsystem  Commented=on
  Terminator : Terminator
  Transfer Fcn : TransferFcn  Numerator=[0.1783]  Denominator=[1 0.0141]
  Transfer Fcn1 : TransferFcn  Numerator=[0.2183 0.0018]  Denominator=[1 0.0283 0.0002]
  Transfer Fcn2 : TransferFcn  Numerator=[0.2884 0.0094]  Denominator=[1 0.1131 0.0032]
  VD : Constant  Value=0
  VE : Constant  Value=2
  VN : Constant  Value=2
  Wind Speed : MATLAB Function  TreatAsAtomicUnit=on
  Out1 : Outport  VectorParamsAs1DForOutWhenUnconnected=off
  wires:
  Transfer Fcn/1 -> Scope1/1, Add/1
  VD/1 -> Mux/3
  Mux/1 -> Wind Speed/1(uu)
  Wind Speed/3(v) -> Add1/2
  Wind Speed/2(u) -> Add/2
  Band-Limited White Noise2/1 -> Transfer Fcn2/1
  Transfer Fcn2/1 -> Scope2/1, Add2/1
  Band-Limited White Noise1/1 -> Transfer Fcn1/1
  VE/1 -> Mux/2
  Add/1 -> Scope5/1, Mux1/1
  Add1/1 -> Mux1/2, Scope6/1
  Band-Limited White Noise/1 -> Transfer Fcn/1
  Add2/1 -> Mux1/3, Scope7/1
  VN/1 -> Mux/1
  Wind Speed/4(w) -> Add2/2
  Transfer Fcn1/1 -> Scope3/1, Add1/1
  Wind Speed/1(V) -> Terminator/1
  Mux1/1 -> Out1/1

== system Autopilot_q_full_5may_new1/AUTOPILOT /Autopilot Fixed wing mode/Pitch controller ==
  a_z_d : Inport
  Plane_state : Inport  Port=2
  stall_speed : Inport  Port=3
  Aero_coffecients read2 : DataStoreRead  DataStoreName=Aero_cofficients  DataStoreElements=Aero_cofficients(:,:)
  Constant{6..11} (6 alike) : Constant
  Data Store Read : DataStoreRead  DataStoreName=Wind_data  DataStoreElements=Wind_data(:)
  Data Store Read13 : DataStoreRead  DataStoreName=propulsion_model  DataStoreElements=propulsion_model(:)
  Data Store Read15 : DataStoreRead  DataStoreName=Atmospheric_model
  Data Store Read3 : DataStoreRead  DataStoreName=Thrust_data_store  DataStoreElements=Thrust_data_store(:,:)
  Gain{,1..3} (4 alike) : Gain  Gain=57.3
  MATLAB Function1 : MATLAB Function  TreatAsAtomicUnit=on
  MATLAB Function3 : MATLAB Function  TreatAsAtomicUnit=on
  PID Controller (2DOF)2 : simulink/Continuous/PID Controller (2DOF)  Controller=PID  TimeDomain=Discrete-time  SampleTime=0.01  IntegratorMethod=Forward Euler  FilterMethod=Forward Euler  Form=Parallel  UseFilter=on  ControllerParametersSource=internal  P=2.0  I=0.0  D=0  N=100  b=1  c=1  InitialConditionSource=internal  InitialConditionForIntegrator=0  InitialConditionForFilter=0  ExternalReset=none  LimitOutput=off  UpperSaturationLimit=inf  LowerSaturationLimit=-inf  LinearizeAsGain=on  AntiWindupMode=none  Kb=1  TrackingMode=off  Kt=1  PParamMin=[]  PParamMax=[]  IParamMin=[]  IParamMax=[]  DParamMin=[]  DParamMax=[]  NParamMin=[]  NParamMax=[]  bParamMin=[]  bParamMax=[]  cParamMin=[]  cParamMax=[]  KbParamMin=[]  KbParamMax=[]  KtParamMin=[]  KtParamMax=[]  POutMin=[]  POutMax=[]  IOutMin=[]  IOutMax=[]  DOutMin=[]  DOutMax=[]  NOutMin=[]  NOutMax=[]  bOutMin=[]  bOutMax=[]  cOutMin=[]  cOutMax=[]  KbOutMin=[]  KbOutMax=[]  KtOutMin=[]  KtOutMax=[]  IntegratorOutMin=[]  IntegratorOutMax=[]  FilterOutMin=[]  FilterOutMax=[]  SumOutMin=[]  SumOutMax=[]  Sum1OutMin=[]  Sum1OutMax=[]  Sum2OutMin=[]  Sum2OutMax=[]  Sum3OutMin=[]  Sum3OutMax=[]  SumI1OutMin=[]  SumI1OutMax=[]  SumI2OutMin=[]  SumI2OutMax=[]  SumI3OutMin=[]  SumI3OutMax=[]  SumDOutMin=[]  SumDOutMax=[]  SaturationOutMin=[]  SaturationOutMax=[]  IntegratorContinuousStateAttributes=''  IntegratorStateMustResolveToSignalObject=off  IntegratorRTWStateStorageClass=Auto  FilterContinuousStateAttributes=''  FilterStateMustResolveToSignalObject=off  FilterRTWStateStorageClass=Auto  DifferentiatorICPrevScaledInput=0  DifferentiatorOutMin=[]  DifferentiatorOutMax=[]  FilterDiffOutCoefMin=[]  FilterDiffOutCoefMax=[]  SumDenOutMin=[]  SumDenOutMax=[]  SumNumOutMin=[]  SumNumOutMax=[]  ReciprocalOutMin=[]  ReciprocalOutMax=[]  DivideOutMin=[]  DivideOutMax=[]  TunerSelectOption=Transfer Function Based (PID Tuner App)
  PID Controller (2DOF)3 : simulink/Continuous/PID Controller (2DOF)  Controller=PID  TimeDomain=Discrete-time  SampleTime=0.01  IntegratorMethod=Forward Euler  FilterMethod=Forward Euler  Form=Parallel  UseFilter=on  ControllerParametersSource=internal  P=6.0  I=3.0  D=0  N=100  b=1  c=1  InitialConditionSource=internal  InitialConditionForIntegrator=0  InitialConditionForFilter=0  ExternalReset=none  LimitOutput=off  UpperSaturationLimit=inf  LowerSaturationLimit=-inf  LinearizeAsGain=on  AntiWindupMode=none  Kb=1  TrackingMode=off  Kt=1  PParamMin=[]  PParamMax=[]  IParamMin=[]  IParamMax=[]  DParamMin=[]  DParamMax=[]  NParamMin=[]  NParamMax=[]  bParamMin=[]  bParamMax=[]  cParamMin=[]  cParamMax=[]  KbParamMin=[]  KbParamMax=[]  KtParamMin=[]  KtParamMax=[]  POutMin=[]  POutMax=[]  IOutMin=[]  IOutMax=[]  DOutMin=[]  DOutMax=[]  NOutMin=[]  NOutMax=[]  bOutMin=[]  bOutMax=[]  cOutMin=[]  cOutMax=[]  KbOutMin=[]  KbOutMax=[]  KtOutMin=[]  KtOutMax=[]  IntegratorOutMin=[]  IntegratorOutMax=[]  FilterOutMin=[]  FilterOutMax=[]  SumOutMin=[]  SumOutMax=[]  Sum1OutMin=[]  Sum1OutMax=[]  Sum2OutMin=[]  Sum2OutMax=[]  Sum3OutMin=[]  Sum3OutMax=[]  SumI1OutMin=[]  SumI1OutMax=[]  SumI2OutMin=[]  SumI2OutMax=[]  SumI3OutMin=[]  SumI3OutMax=[]  SumDOutMin=[]  SumDOutMax=[]  SaturationOutMin=[]  SaturationOutMax=[]  IntegratorContinuousStateAttributes=''  IntegratorStateMustResolveToSignalObject=off  IntegratorRTWStateStorageClass=Auto  FilterContinuousStateAttributes=''  FilterStateMustResolveToSignalObject=off  FilterRTWStateStorageClass=Auto  DifferentiatorICPrevScaledInput=0  DifferentiatorOutMin=[]  DifferentiatorOutMax=[]  FilterDiffOutCoefMin=[]  FilterDiffOutCoefMax=[]  SumDenOutMin=[]  SumDenOutMax=[]  SumNumOutMin=[]  SumNumOutMax=[]  ReciprocalOutMin=[]  ReciprocalOutMax=[]  DivideOutMin=[]  DivideOutMax=[]  TunerSelectOption=Transfer Function Based (PID Tuner App)
  Scope : Scope  NumInputPorts=2
  Scope1 : Scope  NumInputPorts=2
  Structure_data_read1 : DataStoreRead  DataStoreName=Structural_data  DataStoreElements=Structural_data(:,:)
  Terminator : Terminator
  alpha : Trigonometry  Operator=atan2
  p,q,r,phi,theta,psi : DataStoreRead  DataStoreName=Plane_state_store  DataStoreElements=Plane_state_store(1,4:9)
  "q " : DataStoreRead  DataStoreName=Plane_state_store  DataStoreElements=Plane_state_store(1,5)
  u : DataStoreRead  DataStoreName=Plane_state_store  DataStoreElements=Plane_state_store(1,1)
  w : DataStoreRead  DataStoreName=Plane_state_store  DataStoreElements=Plane_state_store(1,3)
  q_dot_d : Outport  VectorParamsAs1DForOutWhenUnconnected=off
  wires:
  Aero_coffecients read2/1 -> MATLAB Function3/3(aero_data)
  alpha/1 -> PID Controller (2DOF)2/2, Gain1/1
  PID Controller (2DOF)2/1 -> MATLAB Function1/2(alpha_dot_d)
  MATLAB Function3/1(alpha_d) -> PID Controller (2DOF)2/1, Gain/1
  a_z_d/1 -> MATLAB Function3/1(a_z_d)
  Structure_data_read1/1 -> MATLAB Function3/4(structure_data)
  Data Store Read3/1 -> MATLAB Function3/5(Thrust)
  w/1 -> alpha/1
  u/1 -> alpha/2
  Plane_state/1 -> MATLAB Function3/2(Plane_state)
  "q "/1 -> Gain3/1, PID Controller (2DOF)3/2
  PID Controller (2DOF)3/1 -> q_dot_d/1
  p,q,r,phi,theta,psi/1 -> MATLAB Function1/1(angular_state)
  Gain/1 -> Scope1/1
  Gain1/1 -> Scope1/2
  Gain2/1 -> Scope/1
  MATLAB Function1/1(q_d) -> PID Controller (2DOF)3/1, Gain2/1
  Gain3/1 -> Scope/2
  stall_speed/1 -> Terminator/1
  Data Store Read/1 -> MATLAB Function3/6(Wind_ned)
  Data Store Read13/1 -> MATLAB Function3/7(propulsion_data)
  Data Store Read15/1 -> MATLAB Function3/8(atmos_data)
  Constant6/1 -> MATLAB Function3/9(data2)
  Constant7/1 -> MATLAB Function3/10(data3)
  Constant8/1 -> MATLAB Function3/11(data4)
  Constant9/1 -> MATLAB Function3/12(data5)
  Constant10/1 -> MATLAB Function3/13(data6)
  Constant11/1 -> MATLAB Function3/14(data7)
